simulink model "realim_estados_F"  (R2026a)
settings: Solver=ode4  StopTime=60  FixedStep=1e-3
values from neighbouring files (symbols this model uses):
  A = [0,         1,      0,      0 ... (first row only)    [realim_estados_F.m]
  B = [       0 ... (first row only)    [realim_estados_F.m]
  C = [1,         0,      0,      0 ... (first row only)    [realim_estados_F.m]
  D = [0 ... (first row only)    [realim_estados_F.m]
  F = 1 / (Cd2 * inv(I - Ad2 - Bd2 * K_d) * Bd2)    [realim_estados_F.m]
  K_d = -K_d    [realim_estados_F.m]
  L_d = place(Ad2', Cd2', [l1_z, l2_z, l3_z, l4_z])'    [realim_estados_F.m]
  Ts = 20e-3    (= 0.02)    [realim_estados_F.m]
undefined symbols (not defined in the file or in its folder): Ad2, Bd2, Cd2
settings Model: Creator=Dante P  LastModifiedBy=Dante P

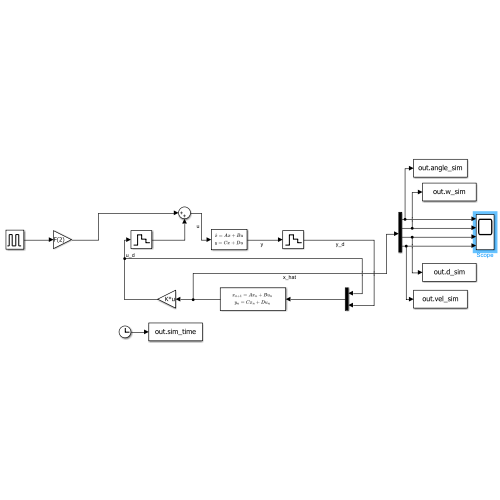
[thumbnail: Simulink's stored preview of the top-level diagram]
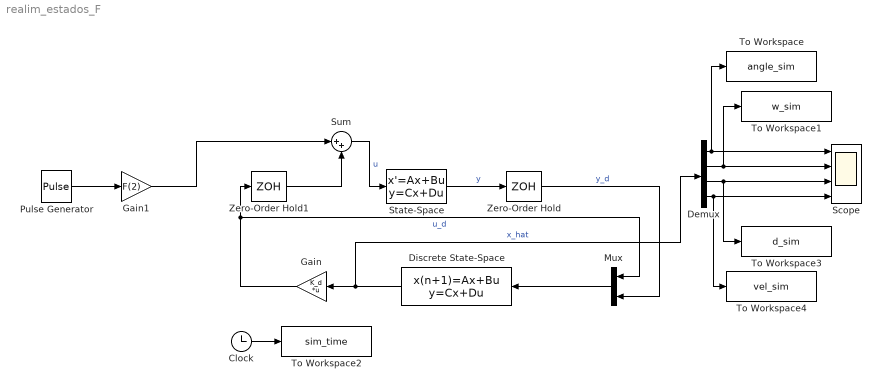
== system realim_estados_F ==
  Clock : Clock
  Demux : Demux
  Discrete State-Space : DiscreteStateSpace  A=Ad2 - L_d * Cd2  B=[Bd2, L_d]  C=eye(4)  D=zeros(4,3)  SampleTime=Ts
  Gain : Gain  Gain=K_d  Multiplication=Matrix(K*u)
  Gain1 : Gain  Gain=F(2)
  Mux : Mux  Inputs=2
  Pulse Generator : DiscretePulseGenerator  PulseType=Time based  Amplitude=8  Period=20  PulseWidth=50
  Scope : Scope  NumInputPorts=4
      settings: ActiveDisplayYMinimum=-61.430794148804637  ActiveDisplayYMaximum=28.646008548277575
  State-Space : StateSpace  A=A  B=B  C=C  D=D  InitialCondition=0
  Sum : Sum  Inputs=|++
  To Workspace : ToWorkspace  VariableName=angle_sim  SampleTime=-1
  To Workspace1 : ToWorkspace  VariableName=w_sim  SampleTime=-1
  To Workspace2 : ToWorkspace  VariableName=sim_time  SampleTime=0.02
  To Workspace3 : ToWorkspace  VariableName=d_sim  SampleTime=-1
  To Workspace4 : ToWorkspace  VariableName=vel_sim  SampleTime=-1
  Zero-Order Hold : ZeroOrderHold  SampleTime=Ts
  Zero-Order Hold1 : ZeroOrderHold  SampleTime=Ts
  wires:
  Gain/1 -> Mux/1, Zero-Order Hold1/1  "u_d"
  Clock/1 -> To Workspace2/1
  State-Space/1 -> Zero-Order Hold/1  "y"
  Discrete State-Space/1 -> Demux/1, Gain/1  "x_hat"
  Zero-Order Hold1/1 -> Sum/2
  Zero-Order Hold/1 -> Mux/2  "y_d"
  Mux/1 -> Discrete State-Space/1
  Demux/1 -> To Workspace/1, Scope/1
  Demux/2 -> To Workspace1/1, Scope/2
  Demux/4 -> To Workspace4/1, Scope/4
  Demux/3 -> To Workspace3/1, Scope/3
  Pulse Generator/1 -> Gain1/1
  Sum/1 -> State-Space/1  "u"
  Gain1/1 -> Sum/1
